simulink model "circuito_RL"  (R2017b)
settings: Solver=VariableStepAuto  StartTime=0.0  StopTime=0.5  RelTol=1e-3
values from neighbouring files (symbols this model uses):
  L = 3    [RL_circuit_data_generator.m]    (also in RL_circuit_data_generator_2.m; gera_dados_circuitoRL.m = 0.001; multi_pinn_data_generation.m)
  omega = 100*rand(1)    [gera_dados_circuitoRL.m]
  R = 3    [RL_circuit_data_generator.m]    (also in RL_circuit_data_generator_2.m; gera_dados_circuitoRL.m = 1000; multi_pinn_data_generation.m)
  v_p = 10*rand(1)    [gera_dados_circuitoRL.m]
settings Model: Creator=Eduardo Rehbein  LastModifiedBy=Eduardo Rehbein

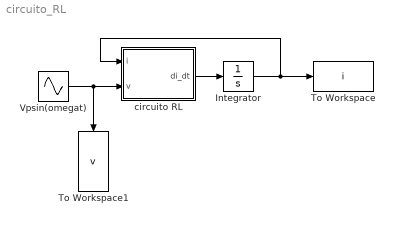
== system circuito_RL ==
  Integrator : Integrator
  To Workspace : ToWorkspace  VariableName=i  SaveFormat=Timeseries  SampleTime=-1
  To Workspace1 : ToWorkspace  VariableName=v  SaveFormat=Timeseries  SampleTime=-1
  Vpsin(omegat) : Sin  Amplitude=v_p  Frequency=omega  SampleTime=0
  circuito RL : MATLAB Function  TreatAsAtomicUnit=on
  wires:
  circuito RL/1(di_dt) -> Integrator/1
  Integrator/1 -> To Workspace/1, circuito RL/1(i)
  Vpsin(omegat)/1 -> circuito RL/2(v), To Workspace1/1

== matlab function circuito_RL/circuito RL ==
  data: i input; di_dt output; v input; R parameter; L parameter
function di_dt = fcn(i, v, R, L)

di_dt = (1/L)*(v - R*i);
